simulink model "robot_hover_final"  (R2016b)
settings: Solver=VariableStepAuto  StartTime=0.0  StopTime=10.0  RelTol=1e-3
values from neighbouring files (symbols this model uses):
  theta_1 = 0.4263    [Untitled_parameters.m]    (also in parametes_pid.m)
  theta_2 = 0.0289    [Untitled_parameters.m]    (also in parametes_pid.m)
  theta_3_1 = theta_3/theta_1    (= 0.0136054421769)    [Untitled_parameters.m]    (also in parametes_pid.m)
  theta_4_1 = theta_4/theta_1    (= 2.31832043162)    [Untitled_parameters.m]    (also in parametes_pid.m)
  theta_5_2 = theta_5/theta_2    (= 0.463667820069)    [Untitled_parameters.m]    (also in parametes_pid.m)
  theta_6_2 = theta_6/theta_2    (= 34.3633217993)    [Untitled_parameters.m]    (also in parametes_pid.m)
libraries: fuzblock x2
settings Model: Creator=asd1  LastModifiedBy=asd1
settings SolverCC: ZeroCrossAlgorithm=Adaptive

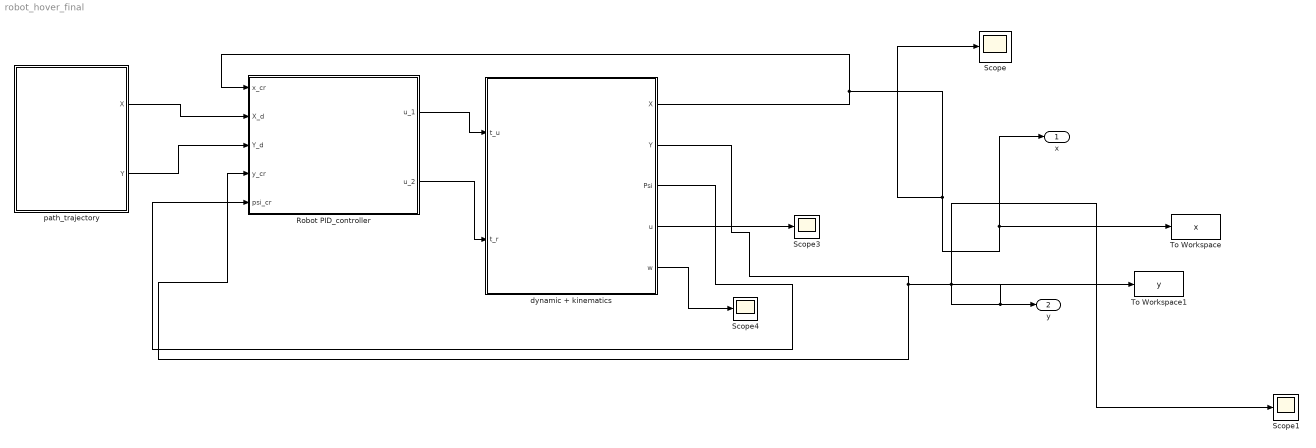
== system robot_hover_final ==
  Robot PID_controller : Subsystem
  Scope{,1,3..4} (4 alike) : Scope
  To Workspace : ToWorkspace  VariableName=x  SampleTime=-1
  To Workspace1 : ToWorkspace  VariableName=y  SampleTime=-1
  "dynamic + kinematics " : Subsystem
  path_trajectory : Subsystem
  x : Outport
  y : Outport  Port=2
  wires:
  "dynamic + kinematics "/1(X) -> To Workspace/1, x/1, Scope/1, Robot PID_controller/1(x_cr)
  "dynamic + kinematics "/2(Y) -> Robot PID_controller/4(y_cr), Scope1/1, To Workspace1/1, y/1
  "dynamic + kinematics "/3(Psi) -> Robot PID_controller/5(psi_cr)
  path_trajectory/1(X) -> Robot PID_controller/2(X_d)
  path_trajectory/2(Y) -> Robot PID_controller/3(Y_d)
  Robot PID_controller/1(u_1) -> "dynamic + kinematics "/1(t_u)
  Robot PID_controller/2(u_2) -> "dynamic + kinematics "/2(t_r)
  "dynamic + kinematics "/4(u) -> Scope3/1
  "dynamic + kinematics "/5(w) -> Scope4/1

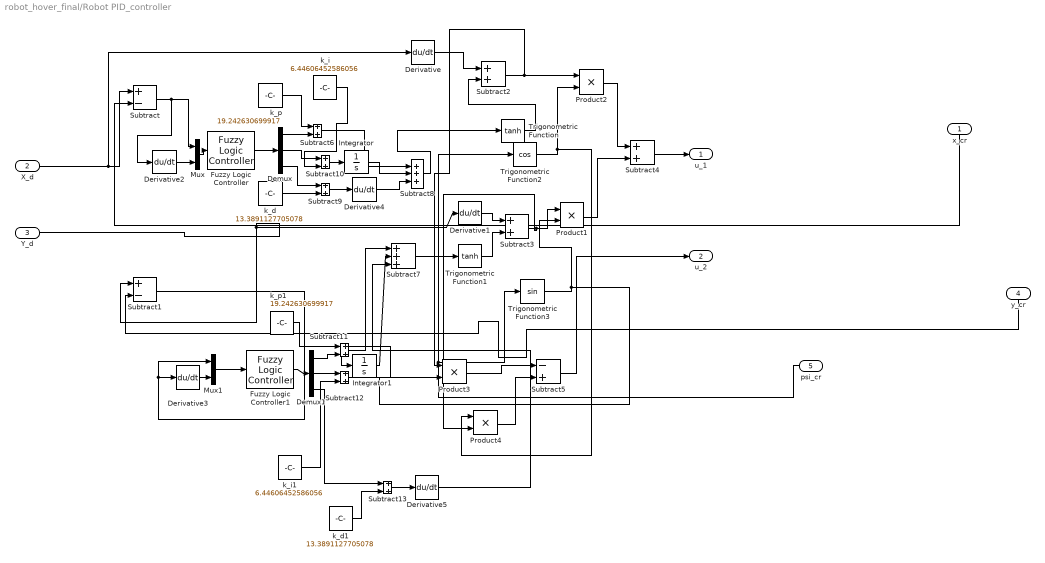
== system robot_hover_final/Robot PID_controller ==
  x_cr : Inport
  X_d : Inport  Port=2
  Y_d : Inport  Port=3
  y_cr : Inport  Port=4
  psi_cr : Inport  Port=5
  Demux : Demux  Outputs=3
  Demux1 : Demux  Outputs=3
  Derivative{,1..5} (6 alike) : Derivative
  Fuzzy Logic Controller : fuzblock/Fuzzy Logic  Controller  fis=optm
  Fuzzy Logic Controller1 : fuzblock/Fuzzy Logic  Controller  fis=optm
  Integrator : Integrator
  Integrator1 : Integrator
  Mux : Mux  Inputs=2
  Mux1 : Mux  Inputs=2
  Product{1..4} (4 alike) : Product
  Subtract : Sum  Inputs=+-
  Subtract1 : Sum  Inputs=+-
  Subtract{2..4,6,9..13} (9 alike) : Sum
  Subtract5 : Sum  Inputs=-+
  Subtract7 : Sum  Inputs=+++
  Subtract8 : Sum  Inputs=+++
  Trigonometric Function : Trigonometry  Operator=tanh
  Trigonometric Function1 : Trigonometry  Operator=tanh
  Trigonometric Function2 : Trigonometry  Operator=cos
  Trigonometric Function3 : Trigonometry
  k_d : Constant  Value=13.3891127705078
  k_d1 : Constant  Value=13.3891127705078
  k_i : Constant  Value=6.44606452586056
  k_i1 : Constant  Value=6.44606452586056
  k_p : Constant  Value=19.242630699917
  k_p1 : Constant  Value=19.242630699917
  u_1 : Outport
  u_2 : Outport  Port=2
  wires:
  Y_d/1 -> Derivative1/1, Subtract1/1
  Subtract/1 -> Derivative2/1, Mux/1
  X_d/1 -> Derivative/1, Subtract/1
  Trigonometric Function/1 -> Subtract2/2
  Derivative/1 -> Subtract2/1
  Trigonometric Function2/1 -> Product4/1, Product2/2
  Subtract1/1 -> Derivative3/1, Mux1/1
  Product4/1 -> Subtract5/2
  Derivative1/1 -> Subtract3/1
  Trigonometric Function1/1 -> Subtract3/2
  Product1/1 -> Subtract4/2
  Subtract2/1 -> Product3/1, Product2/1
  Subtract5/1 -> u_2/1
  Trigonometric Function3/1 -> Product3/2, Product1/2
  Product3/1 -> Subtract5/1
  Product2/1 -> Subtract4/1
  Subtract3/1 -> Product4/2, Product1/1
  psi_cr/1 -> Trigonometric Function3/1, Trigonometric Function2/1
  y_cr/1 -> Subtract1/2
  x_cr/1 -> Subtract/2
  Subtract4/1 -> u_1/1
  Mux/1 -> Fuzzy Logic Controller/1
  Derivative2/1 -> Mux/2
  Mux1/1 -> Fuzzy Logic Controller1/1
  Subtract7/1 -> Trigonometric Function1/1
  Derivative3/1 -> Mux1/2
  Fuzzy Logic Controller/1 -> Demux/1
  Demux/1 -> Subtract6/2
  k_p/1 -> Subtract6/1
  Demux/3 -> Subtract9/1
  k_d/1 -> Subtract9/2
  Demux/2 -> Subtract10/1
  k_i/1 -> Subtract10/2
  Subtract9/1 -> Derivative4/1
  Derivative4/1 -> Subtract8/3
  Subtract6/1 -> Subtract8/1
  Subtract10/1 -> Integrator/1
  Integrator/1 -> Subtract8/2
  Subtract8/1 -> Trigonometric Function/1
  Fuzzy Logic Controller1/1 -> Demux1/1
  k_p1/1 -> Subtract11/1
  Demux1/1 -> Subtract11/2
  Subtract11/1 -> Subtract7/1
  Demux1/2 -> Subtract12/1
  k_i1/1 -> Subtract12/2
  Subtract12/1 -> Integrator1/1
  Integrator1/1 -> Subtract7/2
  Demux1/3 -> Subtract13/1
  k_d1/1 -> Subtract13/2
  Subtract13/1 -> Derivative5/1
  Derivative5/1 -> Subtract7/3

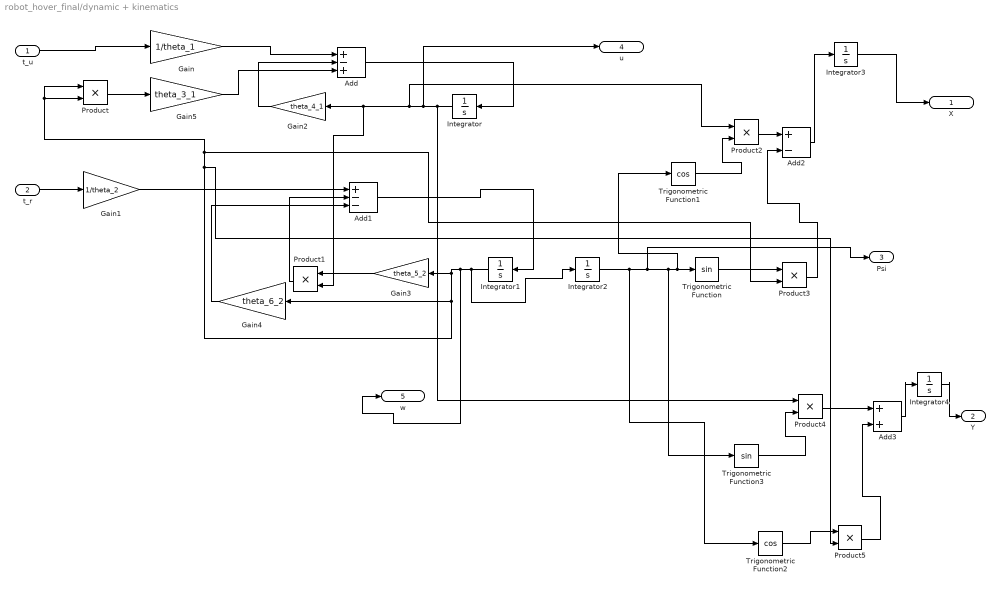
== system robot_hover_final/dynamic + kinematics  ==
  t_u : Inport
  t_r : Inport  Port=2
  Add : Sum  Inputs=+-+
  Add1 : Sum  Inputs=+--
  Add2 : Sum  Inputs=+-
  Add3 : Sum
  Gain : Gain  Gain=1/theta_1
  Gain1 : Gain  Gain=1/theta_2
  Gain2 : Gain  Gain=theta_4_1
  Gain3 : Gain  Gain=theta_5_2
  Gain4 : Gain  Gain=theta_6_2
  Gain5 : Gain  Gain=theta_3_1
  Integrator{,1..4} (5 alike) : Integrator
  Product{,1..5} (6 alike) : Product
  Trigonometric Function : Trigonometry
  Trigonometric Function1 : Trigonometry  Operator=cos
  Trigonometric Function2 : Trigonometry  Operator=cos
  Trigonometric Function3 : Trigonometry
  X : Outport
  Y : Outport  Port=2
  Psi : Outport  Port=3
  u : Outport  Port=4
  w : Outport  Port=5
  wires:
  t_u/1 -> Gain/1
  t_r/1 -> Gain1/1
  Gain/1 -> Add/1
  Add/1 -> Integrator/1
  Integrator/1 -> Product4/1, u/1, Product2/1, Product1/2, Gain2/1
  Gain2/1 -> Add/2
  Gain1/1 -> Add1/1
  Add1/1 -> Integrator1/1
  Integrator1/1 -> Integrator2/1, w/1, Gain4/1, Product5/2, Product3/2, Product/1, Product/2, Gain3/1
  Product/1 -> Gain5/1
  Gain3/1 -> Product1/1
  Product1/1 -> Add1/2
  Gain4/1 -> Add1/3
  Integrator2/1 -> Trigonometric Function2/1, Psi/1, Trigonometric Function3/1, Trigonometric Function1/1, Trigonometric Function/1
  Trigonometric Function1/1 -> Product2/2
  Product2/1 -> Add2/1
  Trigonometric Function/1 -> Product3/1
  Product3/1 -> Add2/2
  Add2/1 -> Integrator3/1
  Trigonometric Function3/1 -> Product4/2
  Product4/1 -> Add3/1
  Trigonometric Function2/1 -> Product5/1
  Product5/1 -> Add3/2
  Add3/1 -> Integrator4/1
  Gain5/1 -> Add/3
  Integrator3/1 -> X/1
  Integrator4/1 -> Y/1

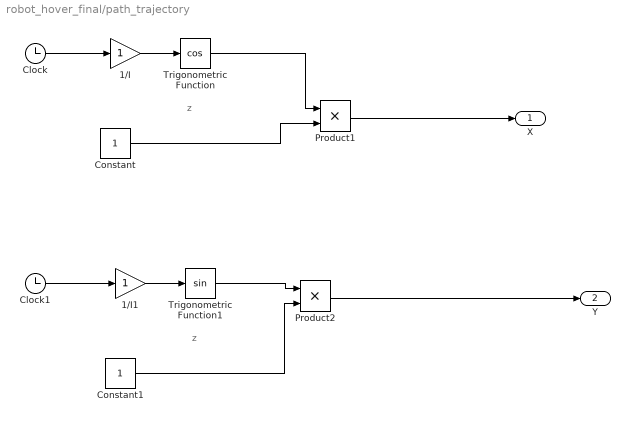
== system robot_hover_final/path_trajectory ==
  note: z
  note: z
  1/I : Gain
  1/I1 : Gain
  Clock : Clock
  Clock1 : Clock
  Constant : Constant
  Constant1 : Constant
  Product1 : Product
  Product2 : Product
  Trigonometric Function : Trigonometry  Operator=cos
  Trigonometric Function1 : Trigonometry
  X : Outport
  Y : Outport  Port=2
  wires:
  1/I/1 -> Trigonometric Function/1
  Constant/1 -> Product1/2
  Trigonometric Function/1 -> Product1/1
  Trigonometric Function1/1 -> Product2/1
  Constant1/1 -> Product2/2
  1/I1/1 -> Trigonometric Function1/1
  Product1/1 -> X/1
  Product2/1 -> Y/1
  Clock1/1 -> 1/I1/1
  Clock/1 -> 1/I/1
